simulink model "Simpel_Model"  (R2016a)
settings: Solver=VariableStepAuto  StartTime=0.0  StopTime=30  RelTol=1e-3
values from neighbouring files (symbols this model uses):
  b = 0.000931    [Model.m]    (also in Projekt_disturbance.m; Rlocus.m = 3.5077e-06)
  D = 1    [PID_test.m]
  I = 4    [PID_test.m]
  J = 0.3    [Model.m]    (also in Projekt_disturbance.m = 0.00567; Rlocus.m = 3.2284e-06)
  K = 651/12    (= 54.25)    [Model.m]    (also in PID_test.m = 96.2958333333; Rlocus.m = 0.0274)
  Kb = 0.509    [Model.m]    (also in Projekt_disturbance.m)
  Km = 0.509    [Model.m]    (also in Projekt_disturbance.m)
  P = 8    [PID_test.m]
  Ra = 7.101    [Model.m]    (also in Projekt_disturbance.m)
  T = 0.014    [Model.m]    (also in PID_test.m = 0.12)
undefined symbols (not defined in the file or in its folder): k
libraries: simulink x1
settings Model: Creator=Kristian  LastModifiedBy=Kristian

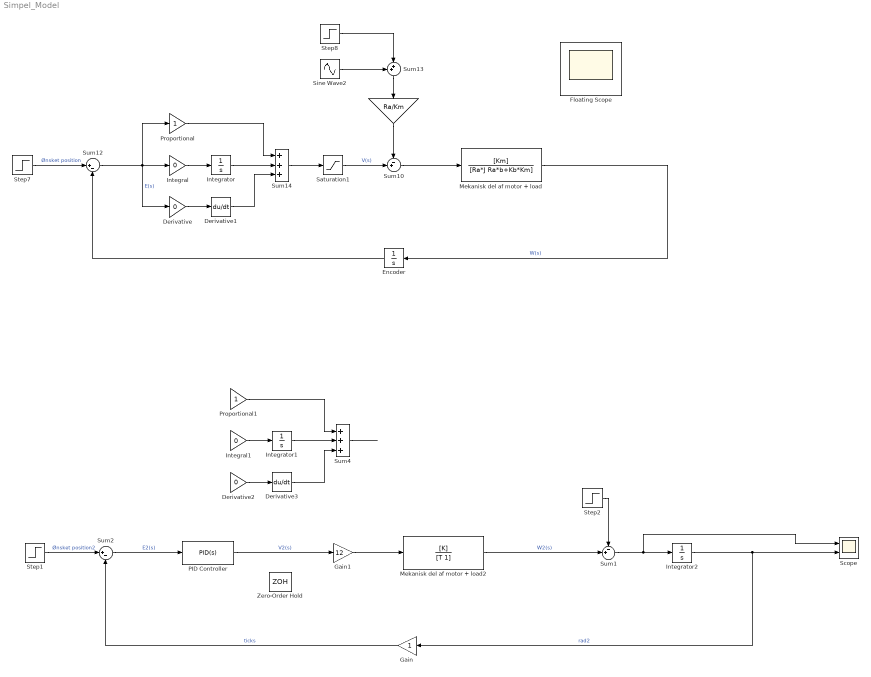
== system Simpel_Model ==
  " " : Gain  Gain=Ra/Km  OutMin=-5  OutMax=5
  Derivative : Gain  Gain=0  OutMin=-5  OutMax=5
  Derivative1 : Derivative
  Derivative2 : Gain  Gain=0  OutMin=-5  OutMax=5
  Derivative3 : Derivative
  "Encoder " : Integrator
  Floating Scope : Scope
      settings: Floating=on
  Gain : Gain
  Gain1 : Gain  Gain=12
  Integral : Gain  Gain=0  OutMin=-5  OutMax=5
  Integral1 : Gain  Gain=0  OutMin=-5  OutMax=5
  Integrator : Integrator
  Integrator1 : Integrator
  Integrator2 : Integrator
  Mekanisk del af motor + load : TransferFcn  Numerator=[Km]  Denominator=[Ra*J Ra*b+Kb*Km]
  Mekanisk del af motor + load2 : TransferFcn  Numerator=[K]  Denominator=[T 1]
  PID Controller : simulink/Continuous/PID Controller  Controller=PID  TimeDomain=Continuous-time  SampleTime=-1  IntegratorMethod=Forward Euler  FilterMethod=Forward Euler  Form=Parallel  UseFilter=off  ControllerParametersSource=internal  P=k*P  I=k*I  D=k*D  N=26.5393027000202  InitialConditionSource=internal  InitialConditionForIntegrator=0  InitialConditionForFilter=0  ExternalReset=none  IgnoreLimit=on  LimitOutput=off  UpperSaturationLimit=1  LowerSaturationLimit=-1  LinearizeAsGain=on  AntiWindupMode=clamping  Kb=1  TrackingMode=off  Kt=1  SaturateOnIntegerOverflow=on  PParamMin=[]  PParamMax=[]  IParamMin=[]  IParamMax=[]  DParamMin=[]  DParamMax=[]  NParamMin=[]  NParamMax=[]  KbParamMin=[]  KbParamMax=[]  KtParamMin=[]  KtParamMax=[]  POutMin=[]  POutMax=[]  IOutMin=[]  IOutMax=[]  DOutMin=[]  DOutMax=[]  NOutMin=[]  NOutMax=[]  KbOutMin=[]  KbOutMax=[]  KtOutMin=[]  KtOutMax=[]  IntegratorOutMin=[]  IntegratorOutMax=[]  FilterOutMin=[]  FilterOutMax=[]  SumOutMin=[]  SumOutMax=[]  SumI1OutMin=[]  SumI1OutMax=[]  SumI2OutMin=[]  SumI2OutMax=[]  SumI3OutMin=[]  SumI3OutMax=[]  SumDOutMin=[]  SumDOutMax=[]  SaturationOutMin=[]  SaturationOutMax=[]  IntegratorContinuousStateAttributes=''  IntegratorStateMustResolveToSignalObject=off  IntegratorRTWStateStorageClass=Auto  FilterContinuousStateAttributes=''  FilterStateMustResolveToSignalObject=off  FilterRTWStateStorageClass=Auto  DifferentiatorICPrevScaledInput=0  DifferentiatorOutMin=[]  DifferentiatorOutMax=[]
  Proportional : Gain  OutMin=-5  OutMax=5
  Proportional1 : Gain  OutMin=-5  OutMax=5
  Saturation1 : Saturate  UpperLimit=12  LowerLimit=-12
  Scope : Scope  NumInputPorts=2
  Sine Wave2 : Sin  Amplitude=0  Frequency=150  SampleTime=0
  Step1 : Step  Time=5  After=2048  SampleTime=0
  Step2 : Step  Time=10  After=20  SampleTime=0
  Step7 : Step  After=10  SampleTime=0
  Step8 : Step  Time=10  After=0.2  SampleTime=0
  Sum1 : Sum  Inputs=-+|
  Sum10 : Sum  Inputs=-+|
  Sum12 : Sum  Inputs=|+-
  Sum13 : Sum  Inputs=++|
  Sum14 : Sum  Inputs=+++
  Sum2 : Sum  Inputs=|+-
  Sum4 : Sum  Inputs=+++
  Zero-Order Hold : ZeroOrderHold  SampleTime=0.0005
  wires:
  Mekanisk del af motor + load/1 -> "Encoder "/1  "W(s)"
  "Encoder "/1 -> Sum12/2
  Sum12/1 -> Derivative/1, Integral/1, Proportional/1  "E(s)"
  Step7/1 -> Sum12/1  "Ønsket position"
  Step8/1 -> Sum13/2
  Sine Wave2/1 -> Sum13/1
  Proportional/1 -> Sum14/1
  Sum14/1 -> Saturation1/1
  Integral/1 -> Integrator/1
  Integrator/1 -> Sum14/2
  Derivative/1 -> Derivative1/1
  Derivative1/1 -> Sum14/3
  Sum10/1 -> Mekanisk del af motor + load/1
  Sum13/1 -> " "/1
  " "/1 -> Sum10/1
  Saturation1/1 -> Sum10/2  "V(s)"
  Gain/1 -> Sum2/2  "ticks"
  Step1/1 -> Sum2/1  "Ønsket position2"
  PID Controller/1 -> Gain1/1  "V2(s)"
  Gain1/1 -> Mekanisk del af motor + load2/1
  ? -> Derivative2/1, Integral1/1, Proportional1/1  "E2(s)"
  Proportional1/1 -> Sum4/1
  Sum4/1 -> ?
  Integral1/1 -> Integrator1/1
  Integrator1/1 -> Sum4/2
  Derivative2/1 -> Derivative3/1
  Derivative3/1 -> Sum4/3
  Sum2/1 -> PID Controller/1  "E2(s)"
  Mekanisk del af motor + load2/1 -> Sum1/2  "W2(s)"
  Sum1/1 -> Scope/1, Integrator2/1
  Step2/1 -> Sum1/1
  Integrator2/1 -> Gain/1, Scope/2  "rad2"
